simulink model "REMUS_OpenLoop_Model"  (R2023a)
settings: Solver=VariableStepAuto  StartTime=0.0  StopTime=2000  FixedStep=0.002  RelTol=1e-3
libraries: simulink x2
settings Model: Creator=邓宇飞  LastModifiedBy=邓宇飞

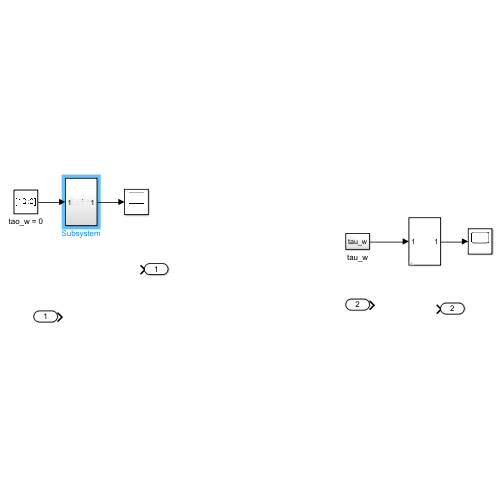
[thumbnail: Simulink's stored preview of the top-level diagram]
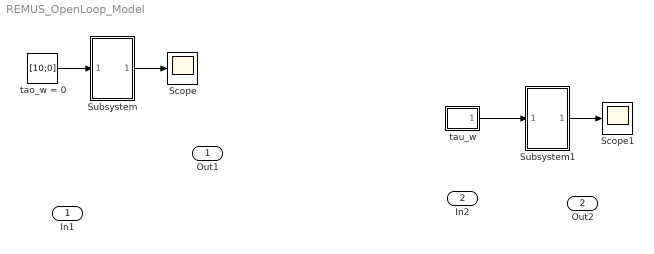
== system REMUS_OpenLoop_Model ==
  In1 : Inport
  In2 : Inport  Port=2
  Scope : Scope
  Scope1 : Scope
  Subsystem : Subsystem
  Subsystem1 : Subsystem
      mask DialogControl ParameterGroupVar Prompt: 参数
  tao_w = 0 : Constant  Value=[10;0]
  tau_w : Subsystem
  Out1 : Outport
  Out2 : Outport  Port=2
  wires:
  tao_w = 0/1 -> Subsystem/1(In1)
  Subsystem/1(Out1) -> Scope/1
  tau_w/1(tau_w) -> Subsystem1/1(In1)
  Subsystem1/1(Out1) -> Scope1/1

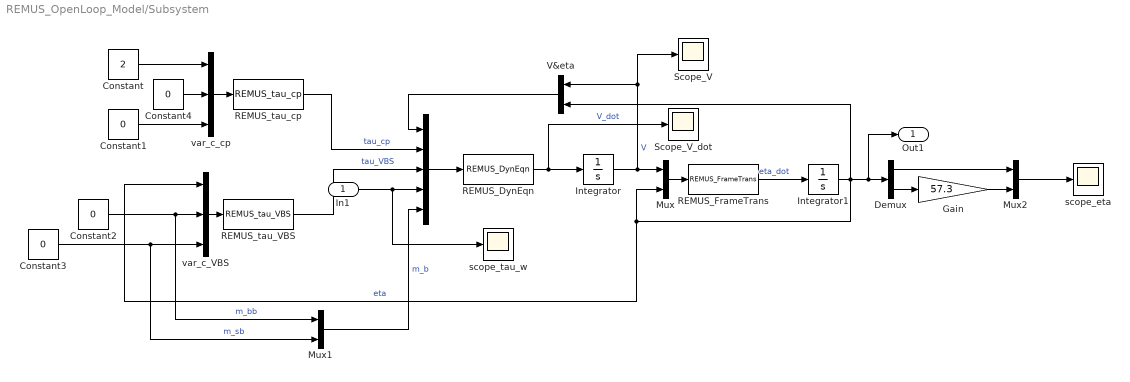
== system REMUS_OpenLoop_Model/Subsystem ==
  In1 : Inport
  " " : Mux  Inputs=5
  Constant : Constant  Value=2
  Constant{1..4} (4 alike) : Constant  Value=0
  Demux : Demux  Outputs=2
  Gain : Gain  Gain=57.3
  Integrator : Integrator
  Integrator1 : Integrator
  Mux : Mux  Inputs=2
  Mux1 : Mux  Inputs=2
  Mux2 : Mux  Inputs=2
  REMUS_DynEqn : MATLABFcn  MATLABFcn=REMUS_DynEqn  OutputDimensions=2
  REMUS_FrameTrans : MATLABFcn  MATLABFcn=REMUS_FrameTrans  OutputDimensions=2
  REMUS_tau_VBS : MATLABFcn  MATLABFcn=REMUS_tau_VBS  OutputDimensions=2
  REMUS_tau_cp : MATLABFcn  MATLABFcn=REMUS_tau_cp  OutputDimensions=2
  Scope_V : Scope
  Scope_V_dot : Scope
  V&eta : Mux  Inputs=2
  scope_eta : Scope
  scope_tau_w : Scope
  var_c_VBS : Mux  Inputs=3
  var_c_cp : Mux  Inputs=3
  Out1 : Outport
  wires:
  Integrator1/1 -> Mux/2, var_c_VBS/1, V&eta/2, Out1/1, Demux/1  "eta"
  Constant2/1 -> var_c_VBS/2, Mux1/1  "m_bb"
  In1/1 -> scope_tau_w/1, " "/4
  " "/1 -> REMUS_DynEqn/1
  Integrator/1 -> Mux/1, V&eta/1, Scope_V/1  "V"
  Constant3/1 -> Mux1/2, var_c_VBS/3  "m_sb"
  REMUS_FrameTrans/1 -> Integrator1/1  "eta_dot"
  REMUS_DynEqn/1 -> Scope_V_dot/1, Integrator/1  "V_dot"
  V&eta/1 -> " "/1
  Constant4/1 -> var_c_cp/2
  var_c_VBS/1 -> REMUS_tau_VBS/1
  REMUS_tau_VBS/1 -> " "/3  "tau_VBS"
  Constant/1 -> var_c_cp/1
  REMUS_tau_cp/1 -> " "/2  "tau_cp"
  Mux1/1 -> " "/5  "m_b"
  Mux/1 -> REMUS_FrameTrans/1
  var_c_cp/1 -> REMUS_tau_cp/1
  Constant1/1 -> var_c_cp/3
  Demux/1 -> Mux2/1
  Demux/2 -> Gain/1
  Mux2/1 -> scope_eta/1
  Gain/1 -> Mux2/2

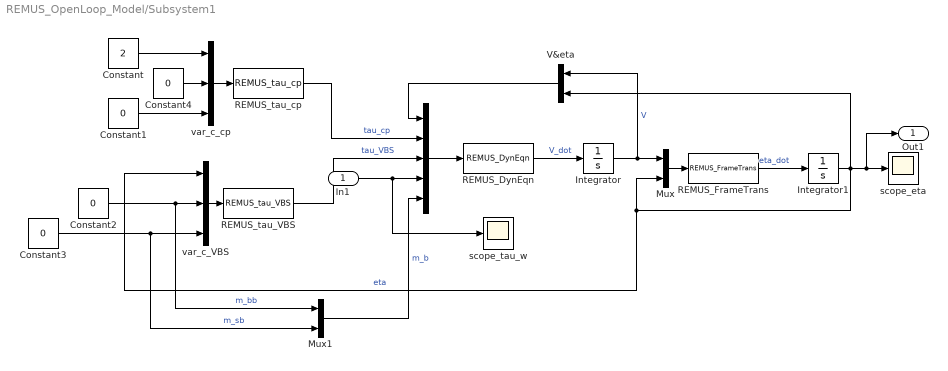
== system REMUS_OpenLoop_Model/Subsystem1 ==
  In1 : Inport
  " " : Mux  Inputs=5
  Constant : Constant  Value=2
  Constant{1..4} (4 alike) : Constant  Value=0
  Integrator : Integrator
  Integrator1 : Integrator
  Mux : Mux  Inputs=2
  Mux1 : Mux  Inputs=2
  REMUS_DynEqn : MATLABFcn  MATLABFcn=REMUS_DynEqn  OutputDimensions=2
  REMUS_FrameTrans : MATLABFcn  MATLABFcn=REMUS_FrameTrans  OutputDimensions=2
  REMUS_tau_VBS : MATLABFcn  MATLABFcn=REMUS_tau_VBS  OutputDimensions=2
  REMUS_tau_cp : MATLABFcn  MATLABFcn=REMUS_tau_cp  OutputDimensions=2
  V&eta : Mux  Inputs=2
  scope_eta : Scope
  scope_tau_w : Scope
  var_c_VBS : Mux  Inputs=3
  var_c_cp : Mux  Inputs=3
  Out1 : Outport
  wires:
  Integrator1/1 -> Mux/2, var_c_VBS/1, V&eta/2, Out1/1, scope_eta/1  "eta"
  Constant2/1 -> var_c_VBS/2, Mux1/1  "m_bb"
  In1/1 -> scope_tau_w/1, " "/4
  " "/1 -> REMUS_DynEqn/1
  Integrator/1 -> Mux/1, V&eta/1  "V"
  Constant3/1 -> Mux1/2, var_c_VBS/3  "m_sb"
  REMUS_FrameTrans/1 -> Integrator1/1  "eta_dot"
  REMUS_DynEqn/1 -> Integrator/1  "V_dot"
  V&eta/1 -> " "/1
  Constant4/1 -> var_c_cp/2
  var_c_VBS/1 -> REMUS_tau_VBS/1
  REMUS_tau_VBS/1 -> " "/3  "tau_VBS"
  Constant/1 -> var_c_cp/1
  REMUS_tau_cp/1 -> " "/2  "tau_cp"
  Mux1/1 -> " "/5  "m_b"
  Mux/1 -> REMUS_FrameTrans/1
  var_c_cp/1 -> REMUS_tau_cp/1
  Constant1/1 -> var_c_cp/3

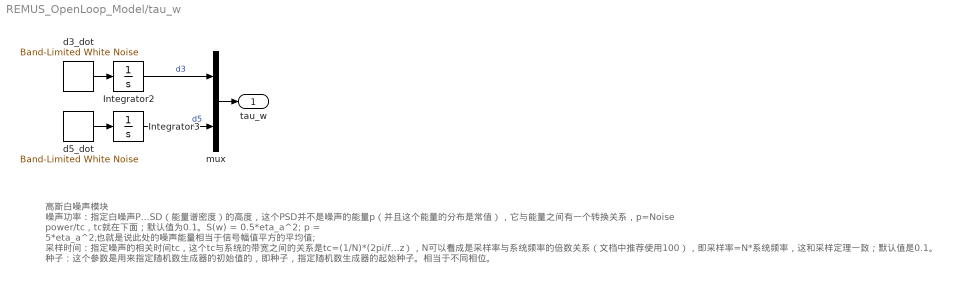
== system REMUS_OpenLoop_Model/tau_w ==
  note: 高斯白噪声模块
      | 噪声功率：指定白噪声PSD（能量谱密度）的高度，这个PSD并不是噪声的能量p（并且这个能量的分布是常值），它与能量之间有一个转换关系，p=Noise power/tc，tc就在下面；默认值为0.1。S(w) = 0.5*eta_a^2;
      | p = 5*eta_a^2;也就是说此处的噪声能量相当于信号幅值平方的平均值;
      | 采样时间：指定噪声的相关时间tc，这个tc与系统的带宽之间的关系是tc=(1/N)*(2pi/fmax)，其中fmax是系统的带宽（实际上是角频率，fmax=2*pi*f，这个f才是我们常使用的频率Hz），N可以看成是采样率与系统频率的倍数关系（文档中推荐使用100），即采样率=N*系统频率，这和采样定理一致；默认值是0.1。
      | 种子：这个参数是用来指定随机数生成器的初始值的，即种子，指定随机数生成器的起始种子。相当于不同相位。
  Integrator2 : Integrator
  Integrator3 : Integrator
  d3_dot : simulink/Sources/Band-Limited White Noise  Cov=[0.5]  Ts=0.1  seed=[2]
  d5_dot : simulink/Sources/Band-Limited White Noise  Cov=[0.1]  Ts=0.1  seed=[3]
  mux : Mux  Inputs=2
  tau_w : Outport
  wires:
  Integrator3/1 -> mux/2  "d5"
  d5_dot/1 -> Integrator3/1
  d3_dot/1 -> Integrator2/1
  mux/1 -> tau_w/1
  Integrator2/1 -> mux/1  "d3"
